simulink model "sistema_1a_ordem_digital_errado"  (R2016b)
settings: Solver=VariableStepAuto  StartTime=0.0  StopTime=50  RelTol=1e-3
settings Model: Creator=fernandopassold  LastModifiedBy=fernandopassold

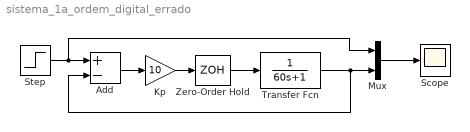
== system sistema_1a_ordem_digital_errado ==
  Add : Sum  Inputs=+-
  Kp : Gain  Gain=10
  Mux : Mux  Inputs=2
  Scope : Scope
  Step : Step  SampleTime=0
  Transfer Fcn : TransferFcn  Denominator=[60 1]
  Zero-Order Hold : ZeroOrderHold  SampleTime=5
  wires:
  Step/1 -> Mux/1, Add/1
  Add/1 -> Kp/1
  Mux/1 -> Scope/1
  Transfer Fcn/1 -> Add/2, Mux/2
  Kp/1 -> Zero-Order Hold/1
  Zero-Order Hold/1 -> Transfer Fcn/1
